simulink model "FlatEarth_MATLAB7VR"  (Simulink 6.6)
settings: Solver=ode45  StartTime=0.0  StopTime=Tstop  RelTol=1e-3
undefined symbols (not defined in the file or in its folder): constant, deltaApertRAD, deltabhppert, deltaEpertRAD, deltaRpertRAD, sigbuilder_block, uIC, Xa, xIC
libraries: aerolibanim x1, vrlib x1
settings Model: Creator=andrisan  LastModifiedBy=andrisan  ExtModeAutoUpdateStatusClock=off
settings DataIOCC: SignalLoggingName=sigsOut
settings OptimizationCC: BooleanDataType=off
settings DebuggingCC: SignalResolutionControl=TryResolveAllWithWarning  SolverPrmCheckMsg=none  MultiTaskDSMMsg=warning  MultiTaskCondExecSysMsg=none  StrictBusMsg=None
settings HardwareCC: TargetUnknown=on
settings RTWCC: IncludeERTFirstTime=on

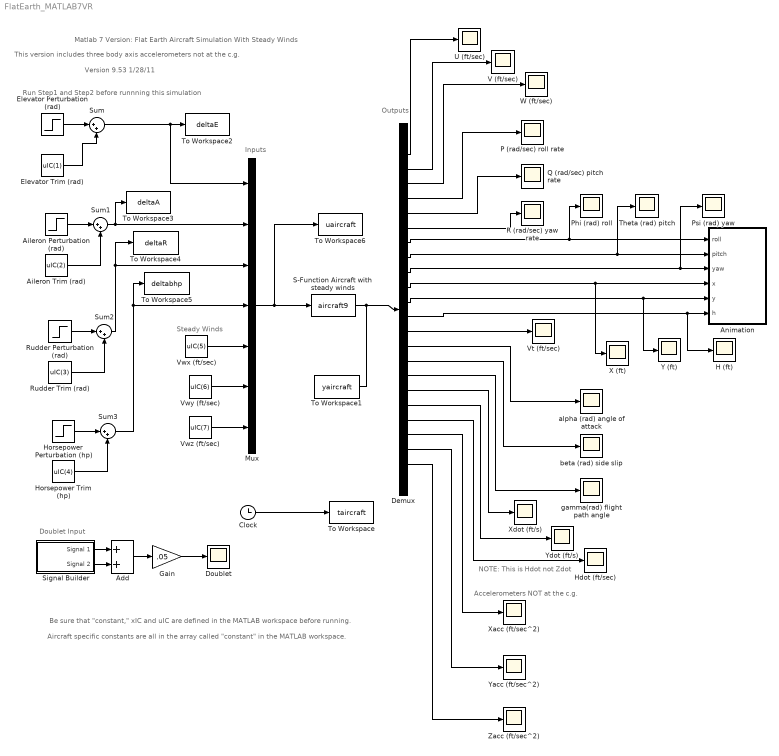
== system FlatEarth_MATLAB7VR ==
  note: Matlab 7 Version: Flat Earth Aircraft Simulation With Steady Winds
  note: Version 9.53 1/28/11
  note: Be sure that "constant," xIC and uIC are defined in the MATLAB workspace before running.
  note: Aircraft specific constants are all in the array called "constant" in the MATLAB workspace.
  note: Steady Winds
  note: Inputs
  note: Outputs
  note: Run Step1 and Step2 before runnning this simulation
  note: This version includes three body axis accelerometers not at the c.g.
  note: Accelerometers NOT at the c.g.
  note: NOTE: This is Hdot not Zdot
  note: Doublet Input
  Add : Sum  OutScaling=2^-10
  Aileron Perturbation (rad) : Step  After=deltaApertRAD  SampleTime=0
  Aileron Trim (rad) : Constant  Value=uIC(2)
  Animation : Subsystem
  Clock : Clock
      settings: Decimation=10
  Demux : Demux  Outputs=22
  Doublet : Scope
      settings: SaveName=ScopeData22
  Elevator Perturbation (rad) : Step  After=deltaEpertRAD  SampleTime=0
  Elevator Trim (rad) : Constant  Value=uIC(1)
  Gain : Gain  Gain=.05
  H (ft) : Scope
      settings: TimeRange=50  SaveName=ScopeData11
  Hdot (ft/sec) : Scope
      settings: SaveName=ScopeData18
  Horsepower Perturbation (hp) : Step  After=deltabhppert  SampleTime=0
  Horsepower Trim (hp) : Constant  Value=uIC(4)
  Mux : Mux  Inputs=7
  P (rad/sec) roll rate : Scope
      settings: SaveName=ScopeData3
  Phi (rad) roll : Scope
      settings: SaveName=ScopeData6
  Psi (rad) yaw : Scope
      settings: SaveName=ScopeData8
  Q (rad/sec) pitch rate : Scope
      settings: SaveName=ScopeData4
  R (rad/sec) yaw rate : Scope
      settings: SaveName=ScopeData5
  Rudder Perturbation (rad) : Step  After=deltaRpertRAD  SampleTime=0
  Rudder Trim (rad) : Constant  Value=uIC(3)
  S-Function Aircraft with  steady winds : S-Function  FunctionName=aircraft9  Parameters=constant,xIC,Xa
  Signal Builder : Subsystem  Tag=STV Subsys  LoadFcn=sigbuilder_block('load');  StartFcn=sigbuilder_block('start');  StopFcn=sigbuilder_block('stop');  ClipboardFcn=sigbuilder_block('clipboard');  mask(Sigbuilder block){}
      mask help: Sigbuilder GUI
      mask init:
      | if ~strcmp(get_param(bdroot(gcbh),'SimulationStatus'),'stopped') tuvar = sigbuilder_block('maskInit'); end
      settings: CopyFcn=sigbuilder_block('copy');  DeleteFcn=sigbuilder_block('delete');  ModelCloseFcn=sigbuilder_block('modelClose');  PreSaveFcn=sigbuilder_block('preSave');  NameChangeFcn=sigbuilder_block('namechange');  OpenFcn=sigbuilder_block('open',[437.6 199.2 550.4 400 ]);  CloseFcn=sigbuilder_block('close');
      mask Display: plot(0,0,100,100,[10,10,40,40,10],[80,20,20,80,80],[40,10],[50,50], [40,27,10],[65,72,56],[40,25,25,10],[28,28,43,43]);
  Sum{,1..3} (4 alike) : Sum  Inputs=|++  SaturateOnIntegerOverflow=on  InputSameDT=on
  Theta (rad) pitch : Scope
      settings: SaveName=ScopeData7
  To Workspace : ToWorkspace  VariableName=taircraft  SampleTime=-1  SaveFormat=Array
  To Workspace1 : ToWorkspace  VariableName=yaircraft  SampleTime=-1  SaveFormat=Array
  To Workspace2 : ToWorkspace  VariableName=deltaE  SampleTime=-1  SaveFormat=Array
  To Workspace3 : ToWorkspace  VariableName=deltaA  SampleTime=-1  SaveFormat=Array
  To Workspace4 : ToWorkspace  VariableName=deltaR  SampleTime=-1  SaveFormat=Array
  To Workspace5 : ToWorkspace  VariableName=deltabhp  SampleTime=-1  SaveFormat=Array
  To Workspace6 : ToWorkspace  VariableName=uaircraft  SampleTime=-1  SaveFormat=Array
  U (ft/sec) : Scope
  V (ft/sec) : Scope
  Vt (ft/sec) : Scope
      settings: TimeRange=50  YMin=99.319  YMax=99.324  SaveName=ScopeData12
  Vwx (ft/sec) : Constant  Value=uIC(5)
  Vwy (ft/sec) : Constant  Value=uIC(6)
  Vwz (ft/sec) : Constant  Value=uIC(7)
  W (ft/sec) : Scope
      settings: YMin=0  YMax=14  SaveName=ScopeData2
  X (ft) : Scope
      settings: SaveName=ScopeData9
  Xacc (ft/sec^2) : Scope
      settings: SaveName=ScopeData19
  Xdot (ft/s) : Scope
      settings: SaveName=ScopeData16
  Y (ft) : Scope
      settings: SaveName=ScopeData10
  Yacc (ft/sec^2) : Scope
      settings: SaveName=ScopeData20
  Ydot (ft/s) : Scope
      settings: SaveName=ScopeData17
  Zacc (ft/sec^2) : Scope
      settings: SaveName=ScopeData21
  alpha (rad) angle of attack : Scope
      settings: SaveName=ScopeData13
  beta (rad) side slip : Scope
      settings: SaveName=ScopeData14
  gamma(rad) flight path angle : Scope
      settings: SaveName=ScopeData15
  wires:
  Demux/1 -> U (ft/sec)/1
  Demux/2 -> V (ft/sec)/1
  Demux/3 -> W (ft/sec)/1
  Demux/4 -> P (rad/sec) roll rate/1
  Demux/5 -> Q (rad/sec) pitch rate/1
  Demux/6 -> R (rad/sec) yaw rate/1
  Demux/8 -> Theta (rad) pitch/1, Animation/2(pitch)
  Demux/9 -> Psi (rad) yaw/1, Animation/3(yaw)
  Demux/10 -> X (ft)/1, Animation/4(x)
  Demux/11 -> Y (ft)/1, Animation/5(y)
  Demux/12 -> H (ft)/1, Animation/6(h)
  Demux/13 -> Vt (ft/sec)/1
  Demux/14 -> alpha (rad) angle of attack/1
  Demux/15 -> beta (rad) side slip/1
  Demux/16 -> gamma(rad) flight path angle/1
  Demux/17 -> Xdot (ft/s)/1
  Demux/18 -> Ydot (ft/s)/1
  Demux/19 -> Hdot (ft/sec)/1
  Clock/1 -> To Workspace/1
  S-Function Aircraft with  steady winds/1 -> Demux/1, To Workspace1/1
  Aileron Perturbation (rad)/1 -> Sum1/1
  Aileron Trim (rad)/1 -> Sum1/2
  Rudder Perturbation (rad)/1 -> Sum2/1
  Rudder Trim (rad)/1 -> Sum2/2
  Horsepower Perturbation (hp)/1 -> Sum3/1
  Horsepower Trim (hp)/1 -> Sum3/2
  Sum/1 -> Mux/1, To Workspace2/1
  Sum1/1 -> Mux/2, To Workspace3/1
  Sum2/1 -> Mux/3, To Workspace4/1
  Sum3/1 -> Mux/4, To Workspace5/1
  Vwx (ft/sec)/1 -> Mux/5
  Vwy (ft/sec)/1 -> Mux/6
  Vwz (ft/sec)/1 -> Mux/7
  Mux/1 -> S-Function Aircraft with  steady winds/1, To Workspace6/1
  Demux/20 -> Xacc (ft/sec^2)/1
  Demux/21 -> Yacc (ft/sec^2)/1
  Demux/22 -> Zacc (ft/sec^2)/1
  Elevator Trim (rad)/1 -> Sum/2
  Add/1 -> Gain/1
  Elevator Perturbation (rad)/1 -> Sum/1
  Gain/1 -> Doublet/1
  Demux/7 -> Animation/1(roll), Phi (rad) roll/1
  Signal Builder/1(Signal 1) -> Add/1
  Signal Builder/2(Signal 2) -> Add/2

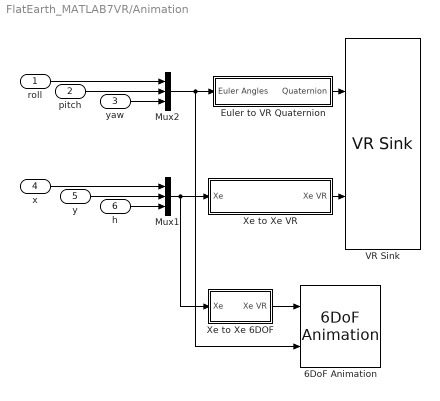
== system FlatEarth_MATLAB7VR/Animation ==
  roll : Inport  OutDataType=fixdt(1,16,0)  OutScaling=[]
  pitch : Inport  Port=2  OutDataType=fixdt(1,16,0)  OutScaling=[]
  yaw : Inport  Port=3  OutDataType=fixdt(1,16,0)  OutScaling=[]
  x : Inport  Port=4  OutDataType=fixdt(1,16,0)  OutScaling=[]
  y : Inport  Port=5  OutDataType=fixdt(1,16,0)  OutScaling=[]
  h : Inport  Port=6  OutDataType=fixdt(1,16,0)  OutScaling=[]
  6DoF Animation : aerolibanim/6DoF Animation  SystemSampleTime=-1  u1=[-10000 10000 -10000 10000 -10000 0]  u2=0.1  u3=20  u4=[0 0 0]  u5=Fly alongside  u6=[100 100 -100]  u7=70  u8=on
  Euler to VR Quaternion : Subsystem
  Mux1 : Mux  Inputs=3
  Mux2 : Mux  Inputs=3
  VR Sink : vrlib/VR Sink  SampleTime=-1  ViewEnable=on  RemoteChange=off  RemoteView=off  FieldsWritten=Plane.rotation.4.1.double#Plane.translation.3.1.double  WorldFileName=F15OverOcean.WRL  AutoView=on  FigureProperties="{'Position', 'Name', 'Viewpoint', 'CameraBound', 'CameraDirection', 'CameraPosition', 'CameraUpVector', 'ZoomFactor', 'Antialiasing', 'Headlight', 'Lighting', 'NavPanel', 'StatusBar', 'ToolBar', 'Textures', 'Transparency', 'Wireframe', 'NavZones', 'NavMode', 'NavSpeed', 'Record2DCompressMethod', 'Record2DCompressQuality', 'Record2D', 'Record2DFileName', 'Record2DFPS'; [1.3300000000000000e+03   6.7000000000000000e+01   5.7600000000000000e+02   3.8000000000000000e+02], '', 'East of Aircraft', 'on', [0.0000000000000000e+00   0.0000000000000000e+00  -1.0000000000000000e+00], [0.0000000000000000e+00   0.0000000000000000e+00   0.0000000000000000e+00], [0.0000000000000000e+00   1.0000000000000000e+00   0.0000000000000000e+00], [1.0000000000000000e+00], 'off', 'on', 'on', 'halfbar', 'on', 'on', 'on', 'on', 'off', 'off', 'walk', 'normal', 'auto', [7.5000000000000000e+01], 'off', '%f_anim_%n.avi', [1.5000000000000000e+01]}"
  Xe to Xe 6DOF : Subsystem
  Xe to Xe VR : Subsystem
  wires:
  Mux2/1 -> Euler to VR Quaternion/1(Euler Angles), 6DoF Animation/2
  Euler to VR Quaternion/1(Quaternion) -> VR Sink/1
  Xe to Xe VR/1(Xe VR) -> VR Sink/2
  Mux1/1 -> Xe to Xe VR/1(Xe), Xe to Xe 6DOF/1(Xe)
  Xe to Xe 6DOF/1(Xe VR) -> 6DoF Animation/1
  roll/1 -> Mux2/1
  pitch/1 -> Mux2/2
  yaw/1 -> Mux2/3
  x/1 -> Mux1/1
  y/1 -> Mux1/2
  h/1 -> Mux1/3

== system FlatEarth_MATLAB7VR/Signal Builder ==
  Demux : Demux  Tag=STV Demux  Outputs=2
  FromWs : FromWorkspace  Tag=STV FromWs  VariableName=tuvar  SampleTime=0  SigBuilderData=DataTag0  VnvData=DataTag1
  Signal 1 : Outport  Tag=STV Outport
  Signal 2 : Outport  Tag=STV Outport  Port=2
  wires:
  Demux/1 -> Signal 1/1
  FromWs/1 -> Demux/1
  Demux/2 -> Signal 2/1

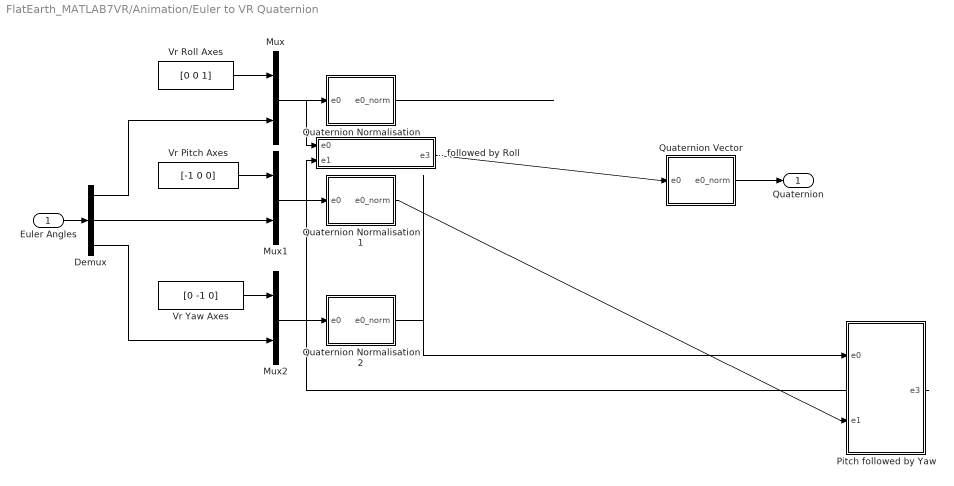
== system FlatEarth_MATLAB7VR/Animation/Euler to VR Quaternion ==
  Euler Angles : Inport
  .. followed by Roll : Subsystem
  Demux : Demux  Outputs=3
  Mux : Mux  Inputs=2
  Mux1 : Mux  Inputs=2
  Mux2 : Mux  Inputs=2
  Pitch followed by Yaw : Subsystem
  Quaternion Normalisation : Subsystem
  Quaternion Normalisation1 : Subsystem
  Quaternion Normalisation2 : Subsystem
  Quaternion Vector : Subsystem
  Vr Pitch Axes : Constant  Value=[-1 0 0]
  Vr Roll Axes : Constant  Value=[0 0 1]
  Vr Yaw Axes : Constant  Value=[0 -1 0]
  Quaternion : Outport
  wires:
  Euler Angles/1 -> Demux/1
  Vr Roll Axes/1 -> Mux/1
  Demux/1 -> Mux/2
  Vr Pitch Axes/1 -> Mux1/1
  Demux/2 -> Mux1/2
  Vr Yaw Axes/1 -> Mux2/1
  Demux/3 -> Mux2/2
  Mux/1 -> Quaternion Normalisation/1(e0)
  Mux1/1 -> Quaternion Normalisation1/1(e0)
  Mux2/1 -> Quaternion Normalisation2/1(e0)
  Quaternion Normalisation1/1(e0_norm) -> Pitch followed by Yaw/2(e1)
  Quaternion Normalisation2/1(e0_norm) -> Pitch followed by Yaw/1(e0)
  Pitch followed by Yaw/1(e3) -> .. followed by Roll/2(e1)
  Quaternion Normalisation/1(e0_norm) -> .. followed by Roll/1(e0)
  .. followed by Roll/1(e3) -> Quaternion Vector/1(e0)
  Quaternion Vector/1(e0_norm) -> Quaternion/1

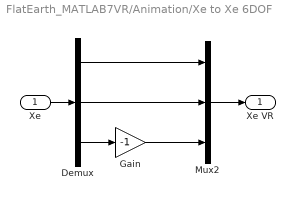
== system FlatEarth_MATLAB7VR/Animation/Xe to Xe 6DOF ==
  Xe : Inport
  Demux : Demux  Outputs=3
  Gain : Gain  Gain=-1
  Mux2 : Mux  Inputs=3
  Xe VR : Outport
  wires:
  Mux2/1 -> Xe VR/1
  Xe/1 -> Demux/1
  Demux/1 -> Mux2/1
  Demux/2 -> Mux2/2
  Demux/3 -> Gain/1
  Gain/1 -> Mux2/3

== system FlatEarth_MATLAB7VR/Animation/Xe to Xe VR ==
  Xe : Inport
  Demux : Demux  Outputs=3
  Mux2 : Mux  Inputs=3
  Xe VR : Outport
  wires:
  Xe/1 -> Demux/1
  Demux/1 -> Mux2/3
  Demux/2 -> Mux2/1
  Demux/3 -> Mux2/2
  Mux2/1 -> Xe VR/1

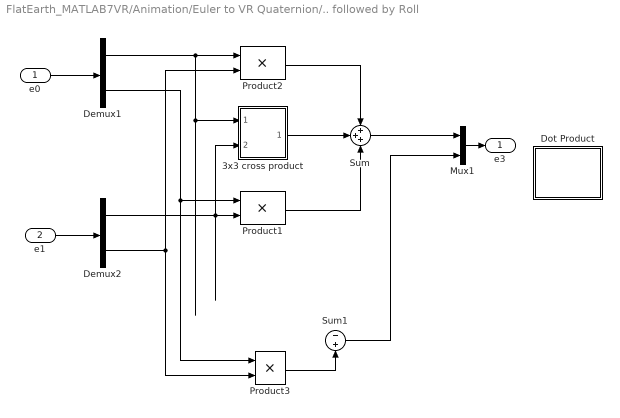
== system FlatEarth_MATLAB7VR/Animation/Euler to VR Quaternion/.. followed by Roll ==
  e0 : Inport
  e1 : Inport  Port=2
  3x3 cross product : Subsystem
      mask Type: Cross Product
      mask Description: Calculates the cross product of two 3x1 vectors.
      mask Help:
      | <p>This block calculates the cross product of two 3x1 vectors, ie.</p>
      | 
      | <ul>C(1) = A(2)*B(3) - A(3)*B(2)</ul>
      | <ul>C(2) = A(3)*B(1) - A(1)*B(3)</ul>
      | <ul>C(3) = A(1)*B(2) - A(2)*B(1)</ul>
      | 
      | <p>The block inputs and output contain more than one signal as described below.</p>
      | 
      | <p><H4>Block Vector Input 1 - A</H4>
      | <ul>
      | <li>A(1)</li>
      | <li>A(2)</li>
      | <li>A(3)</li>
      | </ul>
      | </p>
      | 
      | <p><H4>Block Vector Input 2 - B</H4>
      | <ul>
      | <li>B(1)</li>
      | <li>B(2)</li>
      | <li>B(3)</li>
      | </ul>
      | </p>
      | 
      | <p><H4>Block Vector Output - Cross Product (AxB)</H4>
      | <ul>
      | <li>C(1)</li>
      | <li>C(2)</li>
      | <li>C(3)</li>
      | </ul>
      | </p>
      mask Display: disp('Cross\nProduct')
  Demux1 : Demux  Outputs=[3 1]
  Demux2 : Demux  Outputs=[3 1]
  Dot Product : Subsystem
  Mux1 : Mux  Inputs=2
  Product1 : Product  SaturateOnIntegerOverflow=on  InputSameDT=on
  Product2 : Product  SaturateOnIntegerOverflow=on  InputSameDT=on
  Product3 : Product  SaturateOnIntegerOverflow=on  InputSameDT=on
  Sum : Sum  Inputs=+++  SaturateOnIntegerOverflow=on  InputSameDT=on
  Sum1 : Sum  Inputs=-|+  SaturateOnIntegerOverflow=on  InputSameDT=on
  e3 : Outport
  wires:
  Mux1/1 -> e3/1
  Sum1/1 -> Mux1/2
  Product3/1 -> Sum1/2
  ? -> Sum1/1
  Sum/1 -> Mux1/1
  Product1/1 -> Sum/3
  Product2/1 -> Sum/1
  3x3 cross product/1(c(1) c(2) c(3)) -> Sum/2
  Demux2/2 -> Product3/2, Product2/2
  Demux1/1 -> 3x3 cross product/1(a(1) a(2) a(3)), Product2/1
  Demux2/1 -> 3x3 cross product/2(b(1) b(2) b(3)), Product1/2
  Demux1/2 -> Product3/1, Product1/1
  e1/1 -> Demux2/1
  e0/1 -> Demux1/1

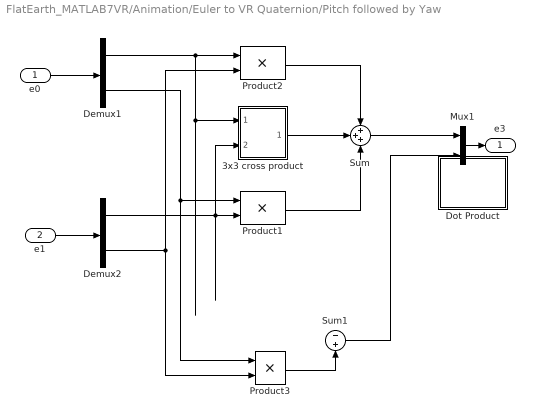
== system FlatEarth_MATLAB7VR/Animation/Euler to VR Quaternion/Pitch followed by Yaw ==
  e0 : Inport
  e1 : Inport  Port=2
  3x3 cross product : Subsystem
      mask Type: Cross Product
      mask Description: Calculates the cross product of two 3x1 vectors.
      mask Help:
      | <p>This block calculates the cross product of two 3x1 vectors, ie.</p>
      | 
      | <ul>C(1) = A(2)*B(3) - A(3)*B(2)</ul>
      | <ul>C(2) = A(3)*B(1) - A(1)*B(3)</ul>
      | <ul>C(3) = A(1)*B(2) - A(2)*B(1)</ul>
      | 
      | <p>The block inputs and output contain more than one signal as described below.</p>
      | 
      | <p><H4>Block Vector Input 1 - A</H4>
      | <ul>
      | <li>A(1)</li>
      | <li>A(2)</li>
      | <li>A(3)</li>
      | </ul>
      | </p>
      | 
      | <p><H4>Block Vector Input 2 - B</H4>
      | <ul>
      | <li>B(1)</li>
      | <li>B(2)</li>
      | <li>B(3)</li>
      | </ul>
      | </p>
      | 
      | <p><H4>Block Vector Output - Cross Product (AxB)</H4>
      | <ul>
      | <li>C(1)</li>
      | <li>C(2)</li>
      | <li>C(3)</li>
      | </ul>
      | </p>
      mask Display: disp('Cross\nProduct')
  Demux1 : Demux  Outputs=[3 1]
  Demux2 : Demux  Outputs=[3 1]
  Dot Product : Subsystem
  Mux1 : Mux  Inputs=2
  Product1 : Product  SaturateOnIntegerOverflow=on  InputSameDT=on
  Product2 : Product  SaturateOnIntegerOverflow=on  InputSameDT=on
  Product3 : Product  SaturateOnIntegerOverflow=on  InputSameDT=on
  Sum : Sum  Inputs=+++  SaturateOnIntegerOverflow=on  InputSameDT=on
  Sum1 : Sum  Inputs=-|+  SaturateOnIntegerOverflow=on  InputSameDT=on
  e3 : Outport
  wires:
  e0/1 -> Demux1/1
  e1/1 -> Demux2/1
  Demux1/2 -> Product1/1, Product3/1
  Demux2/1 -> Product1/2, 3x3 cross product/2(b(1) b(2) b(3))
  Demux1/1 -> Product2/1, 3x3 cross product/1(a(1) a(2) a(3))
  Demux2/2 -> Product2/2, Product3/2
  3x3 cross product/1(c(1) c(2) c(3)) -> Sum/2
  Product2/1 -> Sum/1
  Product1/1 -> Sum/3
  Sum/1 -> Mux1/1
  ? -> Sum1/1
  Product3/1 -> Sum1/2
  Sum1/1 -> Mux1/2
  Mux1/1 -> e3/1

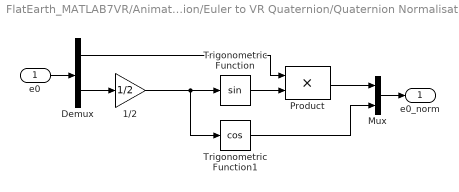
== system FlatEarth_MATLAB7VR/Animation/Euler to VR Quaternion/Quaternion Normalisation ==
  e0 : Inport
  1/2 : Gain  Gain=1/2  SaturateOnIntegerOverflow=on
  Demux : Demux  Outputs=[3 1]
  Mux : Mux  Inputs=2
  Product : Product  SaturateOnIntegerOverflow=on  InputSameDT=on
  Trigonometric Function : Trigonometry
  Trigonometric Function1 : Trigonometry  Operator=cos
  e0_norm : Outport
  wires:
  e0/1 -> Demux/1
  1/2/1 -> Trigonometric Function/1, Trigonometric Function1/1
  Demux/2 -> 1/2/1
  Trigonometric Function/1 -> Product/2
  Demux/1 -> Product/1
  Product/1 -> Mux/1
  Trigonometric Function1/1 -> Mux/2
  Mux/1 -> e0_norm/1

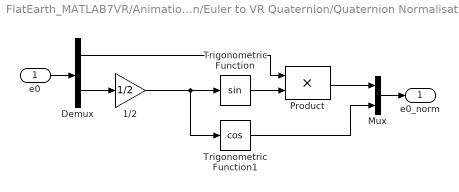
== system FlatEarth_MATLAB7VR/Animation/Euler to VR Quaternion/Quaternion Normalisation1 ==
  e0 : Inport
  1/2 : Gain  Gain=1/2  SaturateOnIntegerOverflow=on
  Demux : Demux  Outputs=[3 1]
  Mux : Mux  Inputs=2
  Product : Product  SaturateOnIntegerOverflow=on  InputSameDT=on
  Trigonometric Function : Trigonometry
  Trigonometric Function1 : Trigonometry  Operator=cos
  e0_norm : Outport
  wires:
  Mux/1 -> e0_norm/1
  Trigonometric Function1/1 -> Mux/2
  Product/1 -> Mux/1
  Demux/1 -> Product/1
  Trigonometric Function/1 -> Product/2
  Demux/2 -> 1/2/1
  1/2/1 -> Trigonometric Function1/1, Trigonometric Function/1
  e0/1 -> Demux/1

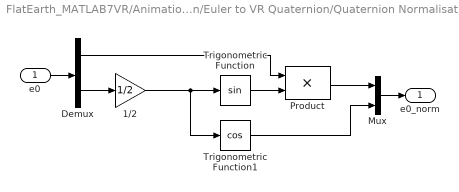
== system FlatEarth_MATLAB7VR/Animation/Euler to VR Quaternion/Quaternion Normalisation2 ==
  e0 : Inport
  1/2 : Gain  Gain=1/2  SaturateOnIntegerOverflow=on
  Demux : Demux  Outputs=[3 1]
  Mux : Mux  Inputs=2
  Product : Product  SaturateOnIntegerOverflow=on  InputSameDT=on
  Trigonometric Function : Trigonometry
  Trigonometric Function1 : Trigonometry  Operator=cos
  e0_norm : Outport
  wires:
  e0/1 -> Demux/1
  1/2/1 -> Trigonometric Function/1, Trigonometric Function1/1
  Demux/2 -> 1/2/1
  Trigonometric Function/1 -> Product/2
  Demux/1 -> Product/1
  Product/1 -> Mux/1
  Trigonometric Function1/1 -> Mux/2
  Mux/1 -> e0_norm/1

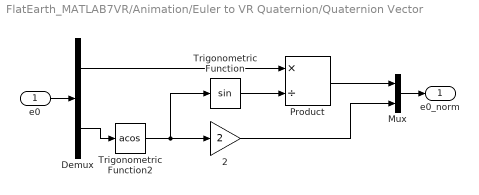
== system FlatEarth_MATLAB7VR/Animation/Euler to VR Quaternion/Quaternion Vector ==
  e0 : Inport
  2 : Gain  Gain=2  SaturateOnIntegerOverflow=on
  Demux : Demux  Outputs=[3 1]
  Mux : Mux  Inputs=2
  Product : Product  Inputs=*/  SaturateOnIntegerOverflow=on  InputSameDT=on
  Trigonometric Function : Trigonometry
  Trigonometric Function2 : Trigonometry  Operator=acos
  e0_norm : Outport
  wires:
  e0/1 -> Demux/1
  Demux/2 -> Trigonometric Function2/1
  Trigonometric Function2/1 -> 2/1, Trigonometric Function/1
  Demux/1 -> Product/1
  Trigonometric Function/1 -> Product/2
  2/1 -> Mux/2
  Product/1 -> Mux/1
  Mux/1 -> e0_norm/1

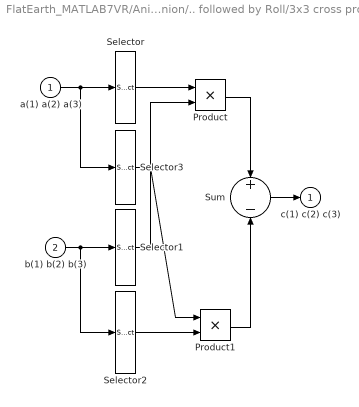
== system FlatEarth_MATLAB7VR/Animation/Euler to VR Quaternion/.. followed by Roll/3x3 cross product ==
  a(1) a(2) a(3) : Inport
  b(1) b(2) b(3) : Inport  Port=2
  Product : Product  SaturateOnIntegerOverflow=on  InputSameDT=on
  Product1 : Product  SaturateOnIntegerOverflow=on  InputSameDT=on
  Selector{,1..3} (4 alike) : Selector  IndexOptions=Index vector (dialog)  Indices=1  OutputSizes=1  InputPortWidth=3
  Sum : Sum  Inputs=+|-  SaturateOnIntegerOverflow=on  InputSameDT=on
  c(1) c(2) c(3) : Outport  InitialOutput=0
  wires:
  Sum/1 -> c(1) c(2) c(3)/1
  b(1) b(2) b(3)/1 -> Selector1/1, Selector2/1
  Selector/1 -> Product/1
  a(1) a(2) a(3)/1 -> Selector/1, Selector3/1
  Product/1 -> Sum/1
  Selector1/1 -> Product/2
  Product1/1 -> Sum/2
  Selector2/1 -> Product1/2
  Selector3/1 -> Product1/1

== system FlatEarth_MATLAB7VR/Animation/Euler to VR Quaternion/.. followed by Roll/Dot Product ==

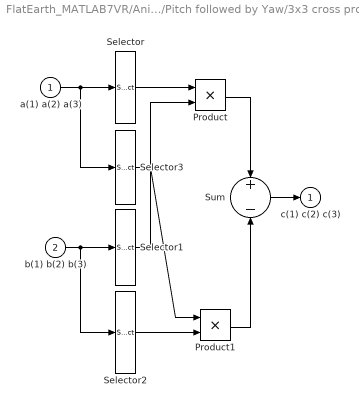
== system FlatEarth_MATLAB7VR/Animation/Euler to VR Quaternion/Pitch followed by Yaw/3x3 cross product ==
  a(1) a(2) a(3) : Inport
  b(1) b(2) b(3) : Inport  Port=2
  Product : Product  SaturateOnIntegerOverflow=on  InputSameDT=on
  Product1 : Product  SaturateOnIntegerOverflow=on  InputSameDT=on
  Selector{,1..3} (4 alike) : Selector  IndexOptions=Index vector (dialog)  Indices=1  OutputSizes=1  InputPortWidth=3
  Sum : Sum  Inputs=+|-  SaturateOnIntegerOverflow=on  InputSameDT=on
  c(1) c(2) c(3) : Outport  InitialOutput=0
  wires:
  Selector3/1 -> Product1/1
  Selector2/1 -> Product1/2
  Product1/1 -> Sum/2
  Selector1/1 -> Product/2
  Product/1 -> Sum/1
  a(1) a(2) a(3)/1 -> Selector3/1, Selector/1
  Selector/1 -> Product/1
  b(1) b(2) b(3)/1 -> Selector2/1, Selector1/1
  Sum/1 -> c(1) c(2) c(3)/1

== system FlatEarth_MATLAB7VR/Animation/Euler to VR Quaternion/Pitch followed by Yaw/Dot Product ==
